simulink model "function_user"  (R2024b)
settings: Solver=VariableStepAuto  StartTime=0.0  StopTime=10.0  RelTol=1e-3
settings Model: Creator=sanja  LastModifiedBy=sanja

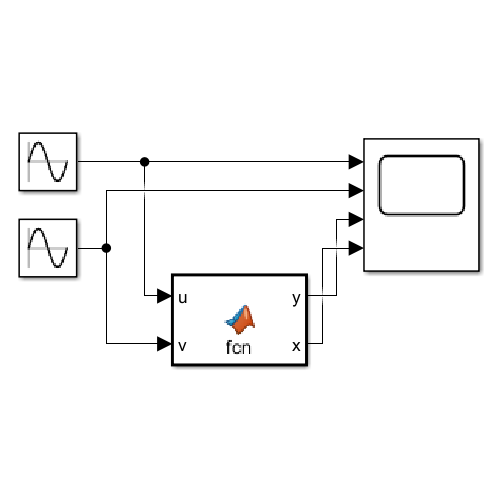
[thumbnail: Simulink's stored preview of the top-level diagram]
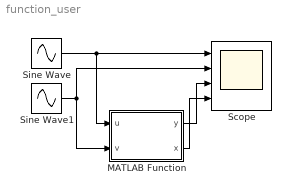
== system function_user ==
  MATLAB Function : MATLAB Function  TreatAsAtomicUnit=on
  Scope : Scope  NumInputPorts=4
  Sine Wave : Sin  Frequency=2  SampleTime=0
  Sine Wave1 : Sin  Frequency=2  Phase=pi/2  SampleTime=0
  wires:
  Sine Wave/1 -> MATLAB Function/1(u), Scope/1
  Sine Wave1/1 -> Scope/2, MATLAB Function/2(v)
  MATLAB Function/1(y) -> Scope/3
  MATLAB Function/2(x) -> Scope/4

== matlab function function_user/MATLAB Function ==
  data: u input; y output; v input; x output
function [y,x] = fcn(u,v)

if u>v
    y = 1
    x = sumfunction(u,v)
else 
    y = 0
    x = 0
end
